simulink model "gm_uz_6ph_pu_vsd_voltages"  (R2021a)
settings: Solver=FixedStepDiscrete  StartTime=0.0  StopTime=64*t_ADC  RelTol=1e-3
undefined symbols (not defined in the file or in its folder): A, f, t_ADC, v_dc, VB
libraries: fl_lib x7, nesl_utility x7, simulink x3, hdlsllib x2, ee_lib x2
settings Model: Creator=micha  LastModifiedBy=micha
settings SolverCC: AlgebraicLoopSolver=TrustRegion
settings DataIOCC: LimitDataPoints=on  SaveOutput=off  SaveTime=off
settings OptimizationCC: BlockReduction=off  ConditionallyExecuteInputs=off  DefaultParameterBehavior=Inlined  LifeSpan=inf
settings DebuggingCC: AlgebraicLoopMsg=error  InheritedTsInSrcMsg=none  SingleTaskRateTransMsg=error  AllowSymbolicDim=off  StrictBusMsg=ErrorOnBusTreatedAsVector  SFUnexpectedBacktrackingDiag=warning  SFNoUnconditionalDefaultTransitionDiag=warning  SFExecutionAtInitializationDiag=none  SFMachineParentedDataDiag=warning  ArithmeticOperatorsInVariantConditions=warning
settings HardwareCC: ProdBitPerPointer=32  ProdBitPerSizeT=32  ProdBitPerPtrDiffT=32  ProdLargestAtomicFloat=None  ProdIntDivRoundTo=Undefined  ProdEndianess=Unspecified  ProdWordSize=32  ProdHWDeviceType=ASIC/FPGA->ASIC/FPGA  ProdEqTarget=off
settings SFSimCC: SimUseLocalCustomCode=off  CustomCodeUndefinedFunction=UseInterfaceOnly
settings RTWCC: RTWUseLocalCustomCode=off
settings CodeAppCC: StateflowObjectComments=on
settings GRTTargetCC: TargetLangStandard=C89/C90 (ANSI)
settings ConfigComp: CovScope=ReferencedModels  CovMetricSettings=dw  CovSaveCumulativeToWorkspaceVar=on  CovSaveSingleToWorkspaceVar=on  CovExternalEMLEnable=off  CovSFcnEnable=off

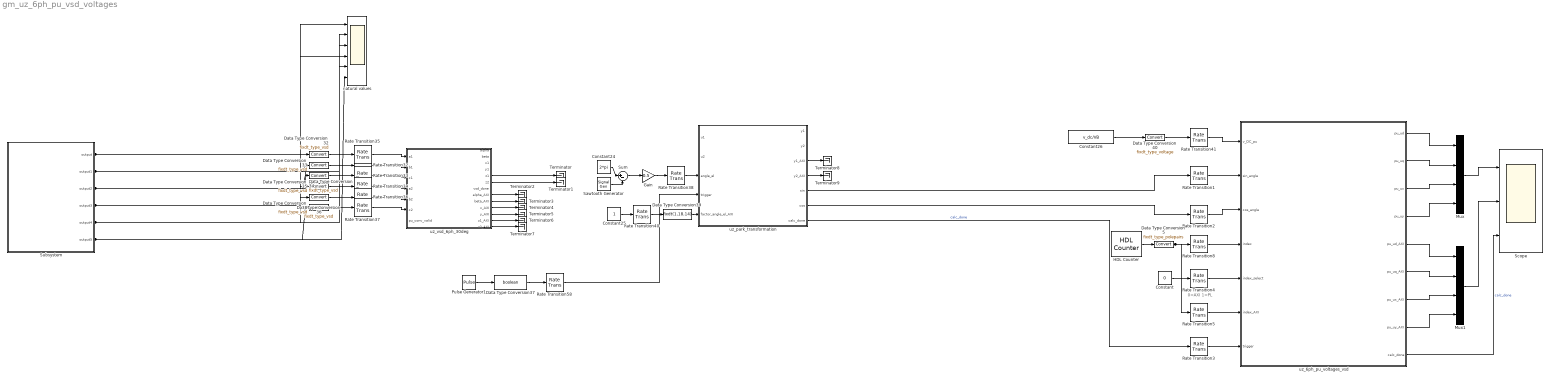
== system gm_uz_6ph_pu_vsd_voltages ==
  note: 0=AXI 1=PL
  Constant : Constant  Value=0  OutDataTypeStr=boolean
  Constant24 : Constant  Value=2*pi
  Constant25 : Constant
  Constant26 : Constant  Value=v_dc/VB
  Data Type Conversion{32..36,38} (6 alike) : DataTypeConversion  OutDataTypeStr=fixdt_type_vsd
  Data Type Conversion37 : DataTypeConversion  OutDataTypeStr=boolean
  Data Type Conversion39 : DataTypeConversion  OutDataTypeStr=fixdt(1,18,14)
  Data Type Conversion40 : DataTypeConversion  OutDataTypeStr=fixdt_type_voltage
  Data Type Conversion5 : DataTypeConversion  OutDataTypeStr=fixdt_type_polepairs
  Gain : Gain  Gain=0.5
  HDL Counter : hdlsllib/Sources/HDL Counter  CountType=Count limited  CountInit=1  CountStep=1  CountMax=64  CountFromType=Initial value  CountFrom=1  CountResetPort=off  CountLoadPort=off  CountEnbPort=off  CountDirPort=off  CountHitOutputPort=off  CountDataType=Unsigned  CountWordLen=8  CountFracLen=0  CountSampTime=t_ADC
  Mux : Mux
  Mux1 : Mux
  Pulse Generator1 : DiscretePulseGenerator  PulseType=Time based  Period=t_ADC  PulseWidth=5
  Rate Transition{1..2,4..5,32..38,40..41,58} (14 alike) : RateTransition  OutPortSampleTime=t_clock
  Rate Transition3 : RateTransition  InitialCondition=1  OutPortSampleTime=t_clock
  Rate Transition8 : RateTransition  InitialCondition=1  OutPortSampleTime=t_clock
  Sawtooth Generator : SignalGenerator  WaveForm=sawtooth  Amplitude=2*pi  Frequency=2*pi*f  Units=rad/sec
  Scope : Scope  NumInputPorts=3
  Subsystem : Subsystem
  Sum : Sum  Inputs=|+-
  Terminator{,1..9} (10 alike) : Terminator
  natural values : Scope  NumInputPorts=6
  uz_6ph_pu_voltages_vsd : Subsystem  TreatAsAtomicUnit=on
  uz_park_transformation : Subsystem  TreatAsAtomicUnit=on
  uz_vsd_6ph_30deg : Subsystem  TreatAsAtomicUnit=on
  wires:
  uz_6ph_pu_voltages_vsd/6(pu_uq_AXI) -> Mux1/2
  uz_6ph_pu_voltages_vsd/7(pu_ux_AXI) -> Mux1/3
  uz_6ph_pu_voltages_vsd/8(pu_uy_AXI) -> Mux1/4
  uz_6ph_pu_voltages_vsd/5(pu_ud_AXI) -> Mux1/1
  Mux1/1 -> Scope/2
  Constant/1 -> Rate Transition4/1
  Rate Transition5/1 -> uz_6ph_pu_voltages_vsd/6(index_AXI)
  Rate Transition4/1 -> uz_6ph_pu_voltages_vsd/5(index_select)
  Rate Transition38/1 -> uz_park_transformation/3(angle_el)
  HDL Counter/1 -> Data Type Conversion5/1
  uz_6ph_pu_voltages_vsd/9(calc_done) -> Scope/3  "calc_done"
  Mux/1 -> Scope/1
  uz_6ph_pu_voltages_vsd/4(pu_uy) -> Mux/4
  uz_6ph_pu_voltages_vsd/3(pu_ux) -> Mux/3
  uz_6ph_pu_voltages_vsd/2(pu_uq) -> Mux/2
  uz_6ph_pu_voltages_vsd/1(pu_ud) -> Mux/1
  uz_park_transformation/7(calc_done) -> Rate Transition3/1  "calc_done"
  Rate Transition3/1 -> uz_6ph_pu_voltages_vsd/7(trigger)
  Pulse Generator1/1 -> Data Type Conversion37/1
  Rate Transition58/1 -> uz_park_transformation/4(trigger)
  Data Type Conversion37/1 -> Rate Transition58/1
  Rate Transition2/1 -> uz_6ph_pu_voltages_vsd/3(cos_angle)
  Rate Transition1/1 -> uz_6ph_pu_voltages_vsd/2(sin_angle)
  uz_park_transformation/6(cos) -> Rate Transition2/1
  uz_park_transformation/5(sin) -> Rate Transition1/1
  uz_vsd_6ph_30deg/13(z2_AXI) -> Terminator7/1
  Data Type Conversion32/1 -> Rate Transition35/1
  uz_park_transformation/4(y2_AXI) -> Terminator9/1
  uz_vsd_6ph_30deg/12(z1_AXI) -> Terminator6/1
  Data Type Conversion36/1 -> Rate Transition36/1
  uz_vsd_6ph_30deg/8(alpha_AXI) -> Terminator2/1
  Rate Transition32/1 -> uz_vsd_6ph_30deg/2(b1)
  uz_park_transformation/3(y1_AXI) -> Terminator8/1
  Subsystem/6(output5) -> Data Type Conversion38/1, natural values/6
  uz_vsd_6ph_30deg/11(y_AXI) -> Terminator5/1
  Subsystem/1(output) -> Data Type Conversion32/1, natural values/1
  Constant24/1 -> Sum/1
  Rate Transition36/1 -> uz_vsd_6ph_30deg/5(b2)
  Rate Transition35/1 -> uz_vsd_6ph_30deg/1(a1)
  Data Type Conversion33/1 -> Rate Transition32/1
  Data Type Conversion38/1 -> Rate Transition37/1
  Subsystem/2(output1) -> Data Type Conversion33/1, natural values/2
  Subsystem/3(output2) -> natural values/3, Data Type Conversion34/1
  Data Type Conversion39/1 -> uz_park_transformation/5(factor_angle_el_AXI)
  uz_vsd_6ph_30deg/10(x_AXI) -> Terminator4/1
  uz_vsd_6ph_30deg/6(z2) -> Terminator1/1
  Rate Transition37/1 -> uz_vsd_6ph_30deg/6(c2)
  Rate Transition34/1 -> uz_vsd_6ph_30deg/4(a2)
  uz_vsd_6ph_30deg/9(beta_AXI) -> Terminator3/1
  Rate Transition33/1 -> uz_vsd_6ph_30deg/3(c1)
  Subsystem/5(output4) -> natural values/5, Data Type Conversion36/1
  Sum/1 -> Gain/1
  Subsystem/4(output3) -> natural values/4, Data Type Conversion35/1
  Gain/1 -> Rate Transition38/1
  Data Type Conversion34/1 -> Rate Transition33/1
  Constant25/1 -> Rate Transition40/1
  Sawtooth Generator/1 -> Sum/2
  Rate Transition40/1 -> Data Type Conversion39/1
  uz_vsd_6ph_30deg/5(z1) -> Terminator/1
  Data Type Conversion35/1 -> Rate Transition34/1
  Data Type Conversion40/1 -> Rate Transition41/1
  Rate Transition41/1 -> uz_6ph_pu_voltages_vsd/1(v_DC_pu)
  Constant26/1 -> Data Type Conversion40/1
  Rate Transition8/1 -> uz_6ph_pu_voltages_vsd/4(index)
  Data Type Conversion5/1 -> Rate Transition5/1, Rate Transition8/1

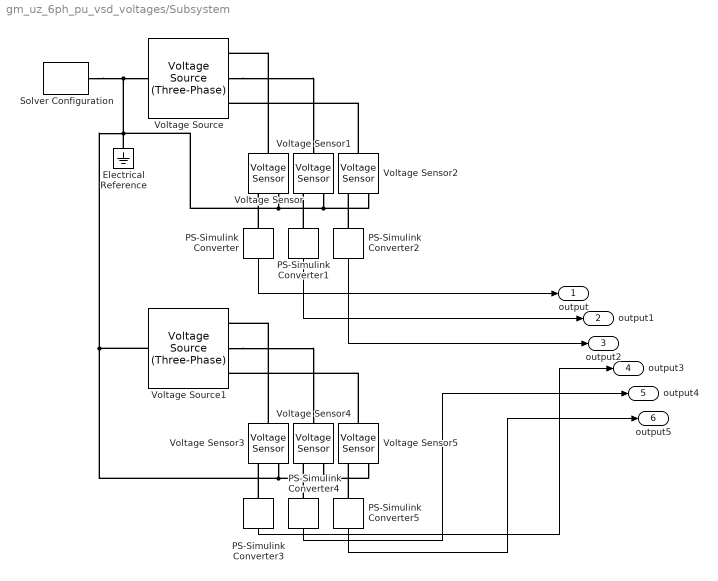
== system gm_uz_6ph_pu_vsd_voltages/Subsystem ==
  Electrical Reference : fl_lib/Electrical/Electrical Elements/Electrical Reference
  PS-Simulink Converter{,1..5} (6 alike) : nesl_utility/PS-Simulink Converter  PhysicalDomain=network_engine_domain  SubClassName=ps_output  LeftPortType=input  RightPortType=output  PseudoPeriodic=off  Frequencies=[]  Unit=1  AffineConversion=off
  Solver Configuration : nesl_utility/Solver Configuration  PhysicalDomain=network_engine_domain  SubClassName=solver  LeftPortType=input  RightPortType=generic  Tones=[]  Harmonics=[]  SimulateNoise=off  Profile=off  UseLocalSampling=off  EnableSwitchedLinearOptims=on  FrequencyDomain=off  UseCCode=off  RelTol=0.001  AbsTol=1e-06  MinStep=1e-09  ToWorkspace=off  RevertToSquareIcSolve=off  NumHomotopyIterations=100  PhasorMode=off  PhasorModeNumHarmonics=1  DoDC=off  ResidualTolerance=1e-09  UseLocalSolver=on  LocalSolverChoice=NE_BACKWARD_EULER_ADVANCER  LocalSolverSampleTime=1e-6  DoFixedCost=on  MaxNonlinIter=3  MaxModeIter=2  ComputeImpulses=off  ImpulseIterations=2  LinearAlgebra=Sparse  EquationFormulation=NE_TIME_EF  DelaysMemoryBudget=1024  AutomaticFiltering=on  FilteringTimeConstant=0.001  PartitionStorageMethod=AS_NEEDED  PartitionMemoryBudget=1024  PartitionMethod=FAST
  Voltage Sensor{,1..5} (6 alike) : fl_lib/Electrical/Electrical Sensors/Voltage Sensor
  Voltage Source : ee_lib/Sources/Voltage Source (Three-Phase)  vline_rms=A*sqrt(3)/sqrt(2) V  shift=0 deg  freq=f Hz  impedance_option=1  SShortCircuit=1e6 V*A  XR=15  R=0.01 Ohm  L=3.97e-4 H  G_parasitic=0 1/Ohm  harmonic_option=1  harmonic_orders=Harmonic_Orders  harmonic_ratios=Harmonic_Amplitudes  I_specify=off  I_priority=None  I=[ 0 0 0 ] A  I_nominal_specify=off  I_nominal_unit=A  I_nominal_value=1
      settings: SourceProductBaseCode=PS  InternalSimscapePortConfiguration="{\"Bottom\":[],\"Left\":[{\"id\":\"n\",\"label\":\"n\",\"type\":\"foundation.electrical.electrical\"}],\"Right\":[{\"id\":\"a\",\"label\":\"a\",\"type\":\"foundation.electrical.electrical\"},{\"id\":\"b\",\"label\":\"b\",\"type\":\"foundation.electrical.electrical\"},{\"id\":\"c\",\"label\":\"c\",\"type\":\"foundation.electrical.electrical\"}],\"Top\":[]}"
  Voltage Source1 : ee_lib/Sources/Voltage Source (Three-Phase)  vline_rms=A*sqrt(3)/sqrt(2) V  shift=-30 deg  freq=f Hz  impedance_option=1  SShortCircuit=1e6 V*A  XR=15  R=0.01 Ohm  L=3.97e-4 H  G_parasitic=0 1/Ohm  harmonic_option=1  harmonic_orders=Harmonic_Orders  harmonic_ratios=Harmonic_Amplitudes  I_specify=off  I_priority=None  I=[ 0 0 0 ] A  I_nominal_specify=off  I_nominal_unit=A  I_nominal_value=1
      settings: SourceProductBaseCode=PS  InternalSimscapePortConfiguration="{\"Bottom\":[],\"Left\":[{\"id\":\"n\",\"label\":\"n\",\"type\":\"foundation.electrical.electrical\"}],\"Right\":[{\"id\":\"a\",\"label\":\"a\",\"type\":\"foundation.electrical.electrical\"},{\"id\":\"b\",\"label\":\"b\",\"type\":\"foundation.electrical.electrical\"},{\"id\":\"c\",\"label\":\"c\",\"type\":\"foundation.electrical.electrical\"}],\"Top\":[]}"
  output : Outport
  output1 : Outport  Port=2
  output2 : Outport  Port=3
  output3 : Outport  Port=4
  output4 : Outport  Port=5
  output5 : Outport  Port=6
  wires:
  PS-Simulink Converter2/1 -> output2/1
  PS-Simulink Converter5/1 -> output5/1
  PS-Simulink Converter1/1 -> output1/1
  PS-Simulink Converter4/1 -> output4/1
  PS-Simulink Converter3/1 -> output3/1
  PS-Simulink Converter/1 -> output/1
  connections:
  Voltage Source/RConn2 -- Voltage Sensor1/LConn1
  Voltage Sensor/LConn1 -- Voltage Source/RConn1
  PS-Simulink Converter3/LConn1 -- Voltage Sensor3/RConn1
  PS-Simulink Converter2/LConn1 -- Voltage Sensor2/RConn1
  Voltage Sensor2/LConn1 -- Voltage Source/RConn3
  PS-Simulink Converter4/LConn1 -- Voltage Sensor4/RConn1
  Voltage Sensor5/LConn1 -- Voltage Source1/RConn3
  Voltage Source1/RConn2 -- Voltage Sensor4/LConn1
  PS-Simulink Converter/LConn1 -- Voltage Sensor/RConn1
  Voltage Sensor3/LConn1 -- Voltage Source1/RConn1
  PS-Simulink Converter1/LConn1 -- Voltage Sensor1/RConn1
  PS-Simulink Converter5/LConn1 -- Voltage Sensor5/RConn1
  Voltage Sensor4/RConn2 -- Voltage Sensor3/RConn2 -- Voltage Source1/LConn1 -- Electrical Reference/LConn1 -- Voltage Sensor/RConn2 -- Voltage Sensor1/RConn2 -- Voltage Sensor2/RConn2 -- Voltage Source/LConn1 -- Solver Configuration/RConn1 -- Voltage Sensor5/RConn2

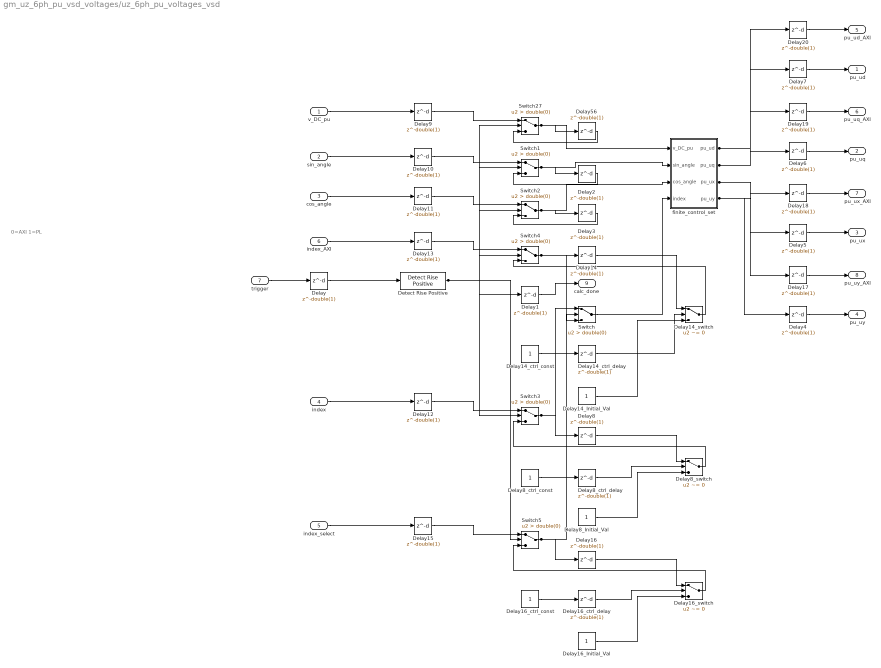
== system gm_uz_6ph_pu_vsd_voltages/uz_6ph_pu_voltages_vsd ==
  note: 0=AXI 1=PL
  v_DC_pu : Inport  OutDataTypeStr=fixdt(1, 18, 15)  PortDimensions=1  SampleTime=1e-08
  sin_angle : Inport  Port=2  OutDataTypeStr=fixdt(1, 18, 16)  PortDimensions=1  SampleTime=1e-08
  cos_angle : Inport  Port=3  OutDataTypeStr=fixdt(1, 18, 16)  PortDimensions=1  SampleTime=1e-08
  index : Inport  Port=4  OutDataTypeStr=uint32  PortDimensions=1  SampleTime=1e-08
  index_select : Inport  Port=5  OutDataTypeStr=boolean  PortDimensions=1  SampleTime=1e-08
  index_AXI : Inport  Port=6  OutDataTypeStr=uint32  PortDimensions=1  SampleTime=1e-08
  trigger : Inport  Port=7  OutDataTypeStr=boolean  PortDimensions=1  SampleTime=1e-08
  Delay{,1..20,56} (22 alike) : Delay  DelayLength=double(1)  InitialCondition=0  SampleTime=1e-08
  Delay14_Initial_Val : Constant  OutDataTypeStr=uint32  SampleTime=1e-08
  Delay14_ctrl_const : Constant  OutDataTypeStr=boolean  SampleTime=1e-08
  Delay14_ctrl_delay : Delay  DelayLength=double(1)  InitialCondition=0  SampleTime=1e-08
  Delay14_switch : Switch  Criteria=u2 ~= 0  Threshold=double(0)  OutDataTypeStr=uint32  SampleTime=1e-08
  Delay16_Initial_Val : Constant  OutDataTypeStr=uint32  SampleTime=1e-08
  Delay16_ctrl_const : Constant  OutDataTypeStr=boolean  SampleTime=1e-08
  Delay16_ctrl_delay : Delay  DelayLength=double(1)  InitialCondition=0  SampleTime=1e-08
  Delay16_switch : Switch  Criteria=u2 ~= 0  Threshold=double(0)  OutDataTypeStr=uint32  SampleTime=1e-08
  Delay8_Initial_Val : Constant  OutDataTypeStr=uint32  SampleTime=1e-08
  Delay8_ctrl_const : Constant  OutDataTypeStr=boolean  SampleTime=1e-08
  Delay8_ctrl_delay : Delay  DelayLength=double(1)  InitialCondition=0  SampleTime=1e-08
  Delay8_switch : Switch  Criteria=u2 ~= 0  Threshold=double(0)  OutDataTypeStr=uint32  SampleTime=1e-08
  Detect Rise Positive : simulink/Logic and Bit Operations/Detect Rise Positive  vinit=0  OutDataTypeStr=boolean
  Switch{,3..5} (4 alike) : Switch  Criteria=u2 > Threshold  Threshold=double(0)  OutDataTypeStr=uint32  SampleTime=1e-08
  Switch1 : Switch  Criteria=u2 > Threshold  Threshold=double(0)  OutDataTypeStr=fixdt(1, 18, 16)  SampleTime=1e-08
  Switch2 : Switch  Criteria=u2 > Threshold  Threshold=double(0)  OutDataTypeStr=fixdt(1, 18, 16)  SampleTime=1e-08
  Switch27 : Switch  Criteria=u2 > Threshold  Threshold=double(0)  OutDataTypeStr=fixdt(1, 18, 15)  SampleTime=1e-08
  finite_control_set : Subsystem
  pu_ud : Outport  SampleTime=1e-08
  pu_uq : Outport  Port=2  SampleTime=1e-08
  pu_ux : Outport  Port=3  SampleTime=1e-08
  pu_uy : Outport  Port=4  SampleTime=1e-08
  pu_ud_AXI : Outport  Port=5  SampleTime=1e-08
  pu_uq_AXI : Outport  Port=6  SampleTime=1e-08
  pu_ux_AXI : Outport  Port=7  SampleTime=1e-08
  pu_uy_AXI : Outport  Port=8  SampleTime=1e-08
  calc_done : Outport  Port=9  SampleTime=1e-08
  wires:
  v_DC_pu/1 -> Delay9/1
  sin_angle/1 -> Delay10/1
  cos_angle/1 -> Delay11/1
  index/1 -> Delay12/1
  index_select/1 -> Delay15/1
  index_AXI/1 -> Delay13/1
  trigger/1 -> Delay/1
  Delay/1 -> Detect Rise Positive/1
  Delay1/1 -> calc_done/1
  Delay10/1 -> Switch1/1
  Delay11/1 -> Switch2/1
  Delay12/1 -> Switch3/1
  Delay13/1 -> Switch4/1
  Delay14_switch/1 -> Switch4/3
  Delay15/1 -> Switch5/1
  Delay16_switch/1 -> Switch5/3
  Delay17/1 -> pu_uy_AXI/1
  Delay18/1 -> pu_ux_AXI/1
  Delay19/1 -> pu_uq_AXI/1
  Delay2/1 -> Switch1/3
  Delay20/1 -> pu_ud_AXI/1
  Delay3/1 -> Switch2/3
  Delay4/1 -> pu_uy/1
  Delay5/1 -> pu_ux/1
  Delay56/1 -> Switch27/3
  Delay6/1 -> pu_uq/1
  Delay7/1 -> pu_ud/1
  Delay8_switch/1 -> Switch3/3
  Delay9/1 -> Switch27/1
  Detect Rise Positive/1 -> Switch5/2, Switch4/2, Switch3/2, Switch27/2, Switch2/2, Switch1/2, Delay1/1
  Switch/1 -> finite_control_set/4(index)
  Switch1/1 -> Delay2/1, finite_control_set/2(sin_angle)
  Switch2/1 -> Delay3/1, finite_control_set/3(cos_angle)
  Switch27/1 -> Delay56/1, finite_control_set/1(v_DC_pu)
  Switch3/1 -> Switch/1, Delay8/1
  Switch4/1 -> Switch/3, Delay14/1
  Switch5/1 -> Switch/2, Delay16/1
  finite_control_set/1(pu_ud) -> Delay7/1, Delay20/1
  finite_control_set/2(pu_uq) -> Delay6/1, Delay19/1
  finite_control_set/3(pu_ux) -> Delay5/1, Delay18/1
  finite_control_set/4(pu_uy) -> Delay4/1, Delay17/1
  Delay14/1 -> Delay14_switch/1
  Delay14_Initial_Val/1 -> Delay14_switch/3
  Delay14_ctrl_const/1 -> Delay14_ctrl_delay/1
  Delay14_ctrl_delay/1 -> Delay14_switch/2
  Delay16/1 -> Delay16_switch/1
  Delay16_Initial_Val/1 -> Delay16_switch/3
  Delay16_ctrl_const/1 -> Delay16_ctrl_delay/1
  Delay16_ctrl_delay/1 -> Delay16_switch/2
  Delay8/1 -> Delay8_switch/1
  Delay8_Initial_Val/1 -> Delay8_switch/3
  Delay8_ctrl_const/1 -> Delay8_ctrl_delay/1
  Delay8_ctrl_delay/1 -> Delay8_switch/2

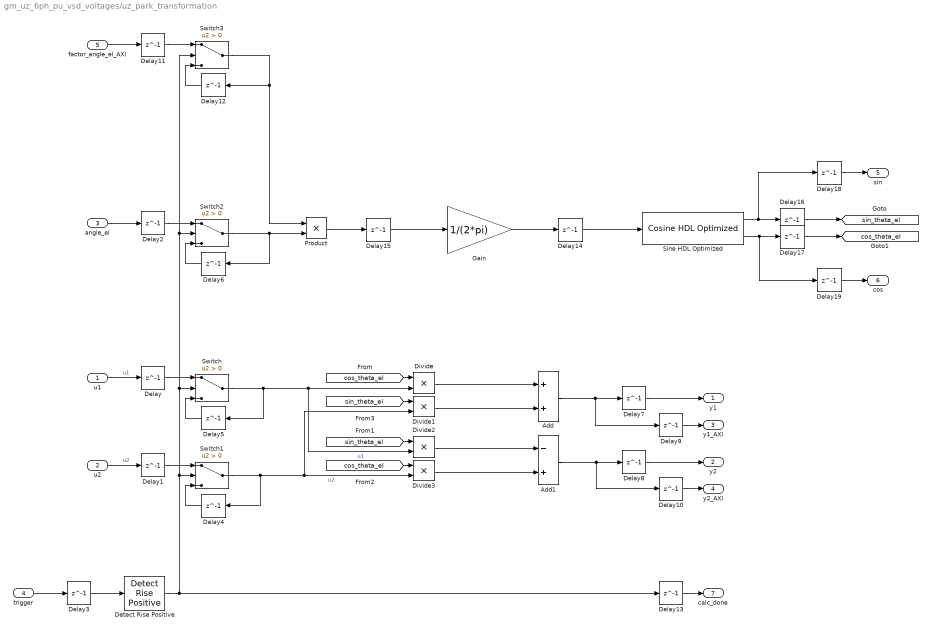
== system gm_uz_6ph_pu_vsd_voltages/uz_park_transformation ==
  u1 : Inport
  u2 : Inport  Port=2
  angle_el : Inport  Port=3
  trigger : Inport  Port=4
  factor_angle_el_AXI : Inport  Port=5
  Add : Sum  OutDataTypeStr=fixdt(1,27,16)
  Add1 : Sum  Inputs=-+  OutDataTypeStr=fixdt(1,27,16)
  Delay{,1..19} (20 alike) : Delay  DelayLength=1
  Detect Rise Positive : simulink/Logic and Bit Operations/Detect Rise Positive  vinit=0  OutDataTypeStr=boolean
  Divide{,1..3} (4 alike) : Product  Inputs=**  OutDataTypeStr=fixdt(1,27,16)
  Gain : Gain  Gain=1/(2*pi)  OutDataTypeStr=fixdt(1,18,16)
  Product : Product  OutDataTypeStr=fixdt(1,18,14)
  Sine HDL Optimized : hdlsllib/Lookup Tables/Cosine HDL Optimized  OutputFormula=sin(2*pi*u) and cos(2*pi*u)  NumDataPoints=256  TableDataTypeStr=fixdt(0,17,16)  SimulateLUTROMDelay=off
      settings: SourceProductBaseCode=SL
  Switch{,1..3} (4 alike) : Switch  Criteria=u2 > Threshold
  y1 : Outport  VectorParamsAs1DForOutWhenUnconnected=off
  y2 : Outport  Port=2  VectorParamsAs1DForOutWhenUnconnected=off
  y1_AXI : Outport  Port=3  VectorParamsAs1DForOutWhenUnconnected=off
  y2_AXI : Outport  Port=4  VectorParamsAs1DForOutWhenUnconnected=off
  sin : Outport  Port=5  VectorParamsAs1DForOutWhenUnconnected=off
  cos : Outport  Port=6  VectorParamsAs1DForOutWhenUnconnected=off
  calc_done : Outport  Port=7  VectorParamsAs1DForOutWhenUnconnected=off
  tag scope: cos_theta_el=global, sin_theta_el=global
  wires:
  Delay19/1 -> cos/1
  Delay18/1 -> sin/1
  Delay17/1 -> [cos_theta_el]
  Delay16/1 -> [sin_theta_el]
  Delay14/1 -> Sine HDL Optimized/1
  Delay15/1 -> Gain/1
  Delay13/1 -> calc_done/1
  Delay3/1 -> Detect Rise Positive/1
  Product/1 -> Delay15/1
  Delay11/1 -> Switch3/1
  Delay12/1 -> Switch3/3
  Detect Rise Positive/1 -> Switch2/2, Switch3/2, Switch/2, Switch1/2, Delay13/1
  factor_angle_el_AXI/1 -> Delay11/1
  Switch3/1 -> Delay12/1, Product/1
  Switch2/1 -> Delay6/1, Product/2
  Delay10/1 -> y2_AXI/1
  Delay9/1 -> y1_AXI/1
  Delay8/1 -> y2/1
  Delay7/1 -> y1/1
  Delay6/1 -> Switch2/3
  Delay5/1 -> Switch/3
  Delay4/1 -> Switch1/3
  trigger/1 -> Delay3/1
  Delay2/1 -> Switch2/1
  Delay1/1 -> Switch1/1
  Delay/1 -> Switch/1
  u2/1 -> Delay1/1  "u2"
  u1/1 -> Delay/1  "u1"
  Gain/1 -> Delay14/1
  Sine HDL Optimized/1 -> Delay16/1, Delay18/1
  Sine HDL Optimized/2 -> Delay17/1, Delay19/1
  angle_el/1 -> Delay2/1
  Divide/1 -> Add/1
  Add1/1 -> Delay8/1, Delay10/1
  Add/1 -> Delay7/1, Delay9/1
  [sin_theta_el] -> Divide1/1
  [cos_theta_el] -> Divide/1
  Divide1/1 -> Add/2
  [sin_theta_el] -> Divide2/1
  Switch/1 -> Delay5/1, Divide/2, Divide2/2  "u1"
  [cos_theta_el] -> Divide3/1
  Divide3/1 -> Add1/2
  Divide2/1 -> Add1/1
  Switch1/1 -> Divide3/2, Divide1/2, Delay4/1  "u2"

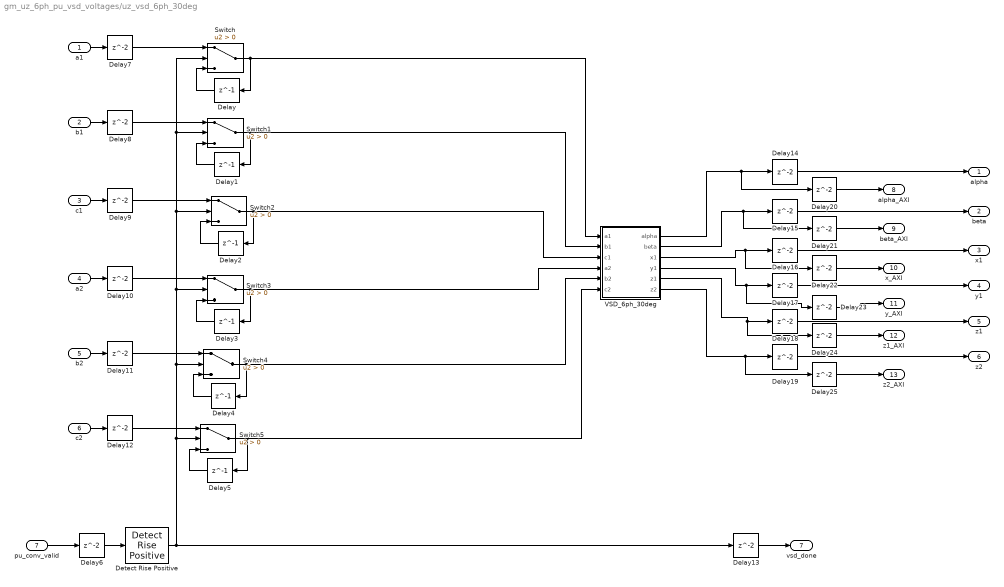
== system gm_uz_6ph_pu_vsd_voltages/uz_vsd_6ph_30deg ==
  a1 : Inport
  b1 : Inport  Port=2
  c1 : Inport  Port=3
  a2 : Inport  Port=4
  b2 : Inport  Port=5
  c2 : Inport  Port=6
  pu_conv_valid : Inport  Port=7
  Delay{,1..5} (6 alike) : Delay  DelayLength=1
  Delay{6..25} (20 alike) : Delay
  Detect Rise Positive : simulink/Logic and Bit Operations/Detect Rise Positive  vinit=0  OutDataTypeStr=boolean
  Switch{,1..5} (6 alike) : Switch  Criteria=u2 > Threshold  OutDataTypeStr=fixdt_type_vsd
  VSD_6ph_30deg : MATLAB Function  TreatAsAtomicUnit=on
  alpha : Outport  OutDataTypeStr=fixdt(1,18,11)  VectorParamsAs1DForOutWhenUnconnected=off
  beta : Outport  Port=2  OutDataTypeStr=fixdt(1,18,11)  VectorParamsAs1DForOutWhenUnconnected=off
  x1 : Outport  Port=3  OutDataTypeStr=fixdt(1,18,11)  VectorParamsAs1DForOutWhenUnconnected=off
  y1 : Outport  Port=4  OutDataTypeStr=fixdt(1,18,11)  VectorParamsAs1DForOutWhenUnconnected=off
  z1 : Outport  Port=5  OutDataTypeStr=fixdt(1,18,11)  VectorParamsAs1DForOutWhenUnconnected=off
  z2 : Outport  Port=6  OutDataTypeStr=fixdt(1,18,11)  VectorParamsAs1DForOutWhenUnconnected=off
  vsd_done : Outport  Port=7  VectorParamsAs1DForOutWhenUnconnected=off
  alpha_AXI : Outport  Port=8  OutDataTypeStr=fixdt(1,18,11)  VectorParamsAs1DForOutWhenUnconnected=off
  beta_AXI : Outport  Port=9  OutDataTypeStr=fixdt(1,18,11)  VectorParamsAs1DForOutWhenUnconnected=off
  x_AXI : Outport  Port=10  OutDataTypeStr=fixdt(1,18,11)  VectorParamsAs1DForOutWhenUnconnected=off
  y_AXI : Outport  Port=11  OutDataTypeStr=fixdt(1,18,11)  VectorParamsAs1DForOutWhenUnconnected=off
  z1_AXI : Outport  Port=12  OutDataTypeStr=fixdt(1,18,11)  VectorParamsAs1DForOutWhenUnconnected=off
  z2_AXI : Outport  Port=13  OutDataTypeStr=fixdt(1,18,11)  VectorParamsAs1DForOutWhenUnconnected=off
  wires:
  Delay25/1 -> z2_AXI/1
  Delay24/1 -> z1_AXI/1
  Delay23/1 -> y_AXI/1
  Delay22/1 -> x_AXI/1
  Delay21/1 -> beta_AXI/1
  Delay20/1 -> alpha_AXI/1
  Delay19/1 -> z2/1
  Delay18/1 -> z1/1
  Delay17/1 -> y1/1
  Delay16/1 -> x1/1
  Delay15/1 -> beta/1
  Delay14/1 -> alpha/1
  Delay13/1 -> vsd_done/1
  Delay12/1 -> Switch5/1
  Delay11/1 -> Switch4/1
  Delay10/1 -> Switch3/1
  Delay9/1 -> Switch2/1
  Delay8/1 -> Switch1/1
  Delay7/1 -> Switch/1
  Delay6/1 -> Detect Rise Positive/1
  c2/1 -> Delay12/1
  b2/1 -> Delay11/1
  a2/1 -> Delay10/1
  c1/1 -> Delay9/1
  b1/1 -> Delay8/1
  a1/1 -> Delay7/1
  Switch5/1 -> Delay5/1, VSD_6ph_30deg/6(c2)
  Delay5/1 -> Switch5/3
  Switch4/1 -> Delay4/1, VSD_6ph_30deg/5(b2)
  Delay4/1 -> Switch4/3
  Switch3/1 -> Delay3/1, VSD_6ph_30deg/4(a2)
  Delay3/1 -> Switch3/3
  Switch2/1 -> Delay2/1, VSD_6ph_30deg/3(c1)
  Delay2/1 -> Switch2/3
  Switch1/1 -> Delay1/1, VSD_6ph_30deg/2(b1)
  Delay1/1 -> Switch1/3
  Switch/1 -> Delay/1, VSD_6ph_30deg/1(a1)
  Delay/1 -> Switch/3
  Detect Rise Positive/1 -> Delay13/1, Switch/2, Switch1/2, Switch2/2, Switch3/2, Switch4/2, Switch5/2
  pu_conv_valid/1 -> Delay6/1
  VSD_6ph_30deg/6(z2) -> Delay19/1, Delay25/1
  VSD_6ph_30deg/5(z1) -> Delay18/1, Delay24/1
  VSD_6ph_30deg/4(y1) -> Delay17/1, Delay23/1
  VSD_6ph_30deg/3(x1) -> Delay16/1, Delay22/1
  VSD_6ph_30deg/2(beta) -> Delay15/1, Delay21/1
  VSD_6ph_30deg/1(alpha) -> Delay14/1, Delay20/1

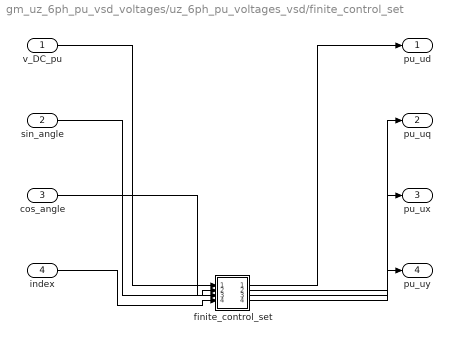
== system gm_uz_6ph_pu_vsd_voltages/uz_6ph_pu_voltages_vsd/finite_control_set ==
  v_DC_pu : Inport  OutDataTypeStr=fixdt(1, 18, 15)  PortDimensions=1  SampleTime=1e-08
  sin_angle : Inport  Port=2  OutDataTypeStr=fixdt(1, 18, 16)  PortDimensions=1  SampleTime=1e-08
  cos_angle : Inport  Port=3  OutDataTypeStr=fixdt(1, 18, 16)  PortDimensions=1  SampleTime=1e-08
  index : Inport  Port=4  OutDataTypeStr=uint32  PortDimensions=1  SampleTime=1e-08
  finite_control_set : MATLAB Function  TreatAsAtomicUnit=on
  pu_ud : Outport  SampleTime=1e-08
  pu_uq : Outport  Port=2  SampleTime=1e-08
  pu_ux : Outport  Port=3  SampleTime=1e-08
  pu_uy : Outport  Port=4  SampleTime=1e-08
  wires:
  v_DC_pu/1 -> finite_control_set/1(v_DC_pu)
  sin_angle/1 -> finite_control_set/2(sin_angle)
  cos_angle/1 -> finite_control_set/3(cos_angle)
  index/1 -> finite_control_set/4(index)
  finite_control_set/1(pu_ud) -> pu_ud/1
  finite_control_set/2(pu_uq) -> pu_uq/1
  finite_control_set/3(pu_ux) -> pu_ux/1
  finite_control_set/4(pu_uy) -> pu_uy/1

== matlab function gm_uz_6ph_pu_vsd_voltages/uz_vsd_6ph_30deg/VSD_6ph_30deg ==
  settings: fimath=fimath('RoundingMethod', 'Floor','OverflowAction', 'Wrap','ProductMode', 'FullPrecision', 'SumMode', 'FullPrecision')
  data: a1 input; alpha output; b1 input; c1 input; a2 input; b2 input; c2 input; beta output; x1 output; y1 output; z1 output; z2 output
function [alpha,beta,x1,y1,z1,z2] = fcn(a1,b1,c1,a2,b2,c2)


A = [fi(0,1,18,11) fi(0,1,18,11) fi(0,1,18,11) fi(0,1,18,11) fi(0,1,18,11) fi(0,1,18,11)]';

A =    2/6*[1    -0.5        -0.5        sqrt(3)/2   -sqrt(3)/2  0 ;
           0    sqrt(3)/2   -sqrt(3)/2  0.5         0.5         -1;
           1    -0.5        -0.5        -sqrt(3)/2  sqrt(3)/2   0 ;
           0    -sqrt(3)/2  sqrt(3)/2   0.5         0.5         -1;
           0.5   0.5          0.5          0           0           0 ;
           0    0           0           0.5          0.5          0.5] * [a1 b1 c1 a2 b2 c2]';

alpha = fi(A(1),1,18,11);
beta = fi(A(2),1,18,11);
x1 = fi(A(3),1,18,11);
y1 = fi(A(4),1,18,11);
z1 = fi(A(5),1,18,11);
z2 = fi(A(6),1,18,11);

== matlab function gm_uz_6ph_pu_vsd_voltages/uz_6ph_pu_voltages_vsd/finite_control_set/finite_control_set ==
  settings: fimath=fimath('RoundingMethod', 'Floor','OverflowAction', 'Wrap','ProductMode', 'FullPrecision', 'SumMode', 'FullPrecision')
  data: v_DC_pu input; sin_angle input; pu_ud output; pu_uq output; pu_ux output; pu_uy output; cos_angle input; index input
function [pu_ud,pu_uq,pu_ux,pu_uy] = voltage_space_vectors(v_DC_pu, sin_angle, cos_angle, index)

fm = fimath();
v_DC_pu = fi(v_DC_pu,1,18,15,fm);
sin_angle = fi(sin_angle,1,18,16,fm);
cos_angle = fi(cos_angle,1,18,16,fm);

% u_d-voltages lookup factors alpha/beta
vd_pu = fi([0.000000,  0.000000;
0.333333,  -0.000000;
-0.166667,  0.288675;
0.166667,  0.288675;
-0.166667,  -0.288675;
0.166667,  -0.288675;
-0.333333,  0.000000;
0.000000,  0.000000;
0.288675,  0.166667;
0.622008,  0.166667;
0.122008,  0.455342;
0.455342,  0.455342;
0.122008,  -0.122008;
0.455342,  -0.122008;
-0.044658,  0.166667;
0.288675,  0.166667;
-0.288675,  0.166667;
0.044658,  0.166667;
-0.455342,  0.455342;
-0.122008,  0.455342;
-0.455342,  -0.122008;
-0.122008,  -0.122008;
-0.622008,  0.166667;
-0.288675,  0.166667;
0.000000,  0.333333;
0.333333,  0.333333;
-0.166667,  0.622008;
0.166667,  0.622008;
-0.166667,  0.044658;
0.166667,  0.044658;
-0.333333,  0.333333;
0.000000,  0.333333;
-0.000000,  -0.333333;
0.333333,  -0.333333;
-0.166667,  -0.044658;
0.166667,  -0.044658;
-0.166667,  -0.622008;
0.166667,  -0.622008;
-0.333333,  -0.333333;
-0.000000,  -0.333333;
0.288675,  -0.166667;
0.622008,  -0.166667;
0.122008,  0.122008;
0.455342,  0.122008;
0.122008,  -0.455342;
0.455342,  -0.455342;
-0.044658,  -0.166667;
0.288675,  -0.166667;
-0.288675,  -0.166667;
0.044658,  -0.166667;
-0.455342,  0.122008;
-0.122008,  0.122008;
-0.455342,  -0.455342;
-0.122008,  -0.455342;
-0.622008,  -0.166667;
-0.288675,  -0.166667;
0.000000,  0.000000;
0.333333,  -0.000000;
-0.166667,  0.288675;
0.166667,  0.288675;
-0.166667,  -0.288675;
0.166667,  -0.288675;
-0.333333,  0.000000;
0.000000,  0.000000],1,18,15);

% u_q-voltages lookup factors alpha/beta
vq_pu = fi([0.000000, 0.000000;
0.333333, -0.000000;
-0.166667, 0.288675;
0.166667, 0.288675;
-0.166667, -0.288675;
0.166667, -0.288675;
-0.333333, 0.000000;
0.000000, 0.000000;
0.288675, 0.166667;
0.622008, 0.166667;
0.122008, 0.455342;
0.455342, 0.455342;
0.122008, -0.122008;
0.455342, -0.122008;
-0.044658, 0.166667;
0.288675, 0.166667;
-0.288675, 0.166667;
0.044658, 0.166667;
-0.455342, 0.455342;
-0.122008, 0.455342;
-0.455342, -0.122008;
-0.122008, -0.122008;
-0.622008, 0.166667;
-0.288675, 0.166667;
0.000000, 0.333333;
0.333333, 0.333333;
-0.166667, 0.622008;
0.166667, 0.622008;
-0.166667, 0.044658;
0.166667, 0.044658;
-0.333333, 0.333333;
0.000000, 0.333333;
-0.000000, -0.333333;
0.333333, -0.333333;
-0.166667, -0.044658;
0.166667, -0.044658;
-0.166667, -0.622008;
0.166667, -0.622008;
-0.333333, -0.333333;
-0.000000, -0.333333;
0.288675, -0.166667;
0.622008, -0.166667;
0.122008, 0.122008;
0.455342, 0.122008;
0.122008, -0.455342;
0.455342, -0.455342;
-0.044658, -0.166667;
0.288675, -0.166667;
-0.288675, -0.166667;
0.044658, -0.166667;
-0.455342, 0.122008;
-0.122008, 0.122008;
-0.455342, -0.455342;
-0.122008, -0.455342;
-0.622008, -0.166667;
-0.288675, -0.166667;
0.000000, 0.000000;
0.333333, -0.000000;
-0.166667, 0.288675;
0.166667, 0.288675;
-0.166667, -0.288675;
0.166667, -0.288675;
-0.333333, 0.000000;
0.000000, 0.000000],1,18,15);
     
% u_x-voltages
vx_pu = fi([0.000000;
0.333333;
-0.166667;
0.166667;
-0.166667;
0.166667;
-0.333333;
0.000000;
-0.288675;
0.044658;
-0.455342;
-0.122008;
-0.455342;
-0.122008;
-0.622008;
-0.288675;
0.288675;
0.622008;
0.122008;
0.455342;
0.122008;
0.455342;
-0.044658;
0.288675;
0.000000;
0.333333;
-0.166667;
0.166667;
-0.166667;
0.166667;
-0.333333;
0.000000;
-0.000000;
0.333333;
-0.166667;
0.166667;
-0.166667;
0.166667;
-0.333333;
-0.000000;
-0.288675;
0.044658;
-0.455342;
-0.122008;
-0.455342;
-0.122008;
-0.622008;
-0.288675;
0.288675;
0.622008;
0.122008;
0.455342;
0.122008;
0.455342;
-0.044658;
0.288675;
0.000000;
0.333333;
-0.166667;
0.166667;
-0.166667;
0.166667;
-0.333333;
0.000000],1,18,15);

% u_y-voltages
vy_pu = fi([0.000000;
-0.000000;
-0.288675;
-0.288675;
0.288675;
0.288675;
0.000000;
0.000000;
0.166667;
0.166667;
-0.122008;
-0.122008;
0.455342;
0.455342;
0.166667;
0.166667;
0.166667;
0.166667;
-0.122008;
-0.122008;
0.455342;
0.455342;
0.166667;
0.166667;
0.333333;
0.333333;
0.044658;
0.044658;
0.622008;
0.622008;
0.333333;
0.333333;
-0.333333;
-0.333333;
-0.622008;
-0.622008;
-0.044658;
-0.044658;
-0.333333;
-0.333333;
-0.166667;
-0.166667;
-0.455342;
-0.455342;
0.122008;
0.122008;
-0.166667;
-0.166667;
-0.166667;
-0.166667;
-0.455342;
-0.455342;
0.122008;
0.122008;
-0.166667;
-0.166667;
0.000000;
-0.000000;
-0.288675;
-0.288675;
0.288675;
0.288675;
0.000000;
0.000000],1,18,15);

pu_ud = fi(v_DC_pu * (vd_pu(index,1) * cos_angle + vd_pu(index,2) * sin_angle),1,27,24);
pu_uq = fi(v_DC_pu * (vq_pu(index,1) * -sin_angle + vq_pu(index,2) * cos_angle),1,27,24);
pu_ux = fi(v_DC_pu * vx_pu(index),1,27,24);
pu_uy = fi(v_DC_pu * vy_pu(index),1,27,24);
